simulink model "Trafo3"  (Simulink 6.5)
settings: Solver=ode23t  StartTime=0.0  StopTime=0.4  RelTol=1e-3
undefined symbols (not defined in the file): D1, Delta, powergui
libraries: powerlib_extras x12, powerlib x11
settings Model: Creator=RS  LastModifiedBy=RS

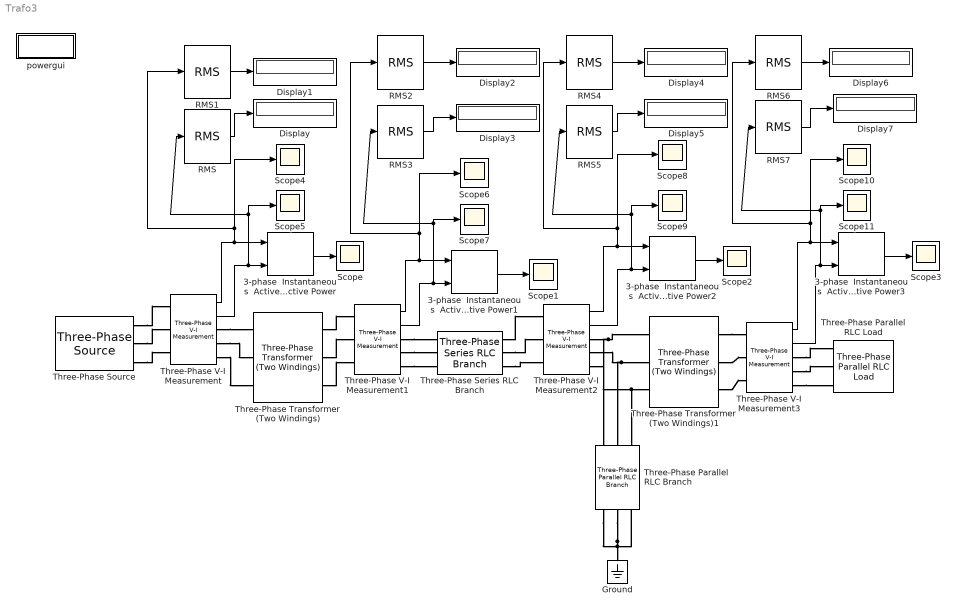
== system Trafo3 ==
  3-phase  Instantaneous  Active & Reactive Power{,1..3} (4 alike) : powerlib_extras/Measurements/3-phase  Instantaneous  Active & Reactive Power  DialogController=PMDialogs.PMDefaultMaskDlg  SystemSampleTime=-1
  Display{,1..7} (8 alike) : Display
  Ground : powerlib/Elements/Ground  Orientation=down  DialogController=PMDialogs.PMDefaultMaskDlg  PhysicalDomain=powersysdomain  SubClassName=unknown  LeftPortType=p1  RightPortType=p1  LConnTagsString=a
  RMS{,1..7} (8 alike) : powerlib_extras/Measurements/RMS  DialogController=PMDialogs.PMDefaultMaskDlg  SystemSampleTime=-1  f1=60
  Scope{,1..11} (12 alike) : Scope
      Scope settings: MaxDataPoints=10000000  SampleInput=on  SampleTime=10e-6
      Scope1 settings: MaxDataPoints=10000000  SampleInput=on  SampleTime=10e-6
      Scope10 settings: SaveName=ScopeData10  MaxDataPoints=10000000  SampleInput=on  SampleTime=10e-6
      Scope11 settings: SaveName=ScopeData11  MaxDataPoints=10000000  SampleInput=on  SampleTime=10e-6
      Scope2 settings: SaveName=ScopeData2  MaxDataPoints=10000000  SampleInput=on  SampleTime=10e-6
      Scope3 settings: YMin=-250000  YMax=3.25e+006  SaveName=ScopeData3  MaxDataPoints=10000000  SampleInput=on  SampleTime=10e-6
      Scope4 settings: SaveName=ScopeData4  MaxDataPoints=10000000  SampleInput=on  SampleTime=10e-6
      Scope5 settings: SaveName=ScopeData5  MaxDataPoints=10000000  SampleInput=on  SampleTime=10e-6
      Scope6 settings: SaveName=ScopeData6  MaxDataPoints=10000000  SampleInput=on  SampleTime=10e-6
      Scope7 settings: SaveName=ScopeData7  MaxDataPoints=10000000  SampleInput=on  SampleTime=10e-6
      Scope8 settings: SaveName=ScopeData8  MaxDataPoints=10000000  SampleInput=on  SampleTime=10e-6
      Scope9 settings: SaveName=ScopeData9  MaxDataPoints=10000000  SampleInput=on  SampleTime=10e-6
  Three-Phase Parallel RLC Branch : powerlib/Elements/Three-Phase Parallel RLC Branch  Orientation=down  DialogController=PMDialogs.PMDefaultMaskDlg  PhysicalDomain=powersysdomain  SubClassName=unknown  LeftPortType=p1  RightPortType=p1  LConnTagsString=A|B|C  RConnTagsString=A|B|C  BranchType=R  Resistance=10000000  Inductance=1e-3  Capacitance=1e-6  Measurements=None
  Three-Phase Parallel RLC Load : powerlib/Elements/Three-Phase Parallel RLC Load  DialogController=PMDialogs.PMDefaultMaskDlg  PhysicalDomain=powersysdomain  SubClassName=unknown  LeftPortType=p1  RightPortType=p1  LConnTagsString=A|B|C  Configuration=Y (grounded)  NominalVoltage=13200  NominalFrequency=60  ActivePower=3000000  InductivePower=0  CapacitivePower=0  Measurements=None
  Three-Phase Series RLC Branch : powerlib/Elements/Three-Phase Series RLC Branch  DialogController=PMDialogs.PMDefaultMaskDlg  PhysicalDomain=powersysdomain  SubClassName=unknown  LeftPortType=p1  RightPortType=p1  LConnTagsString=A|B|C  RConnTagsString=A|B|C  BranchType=RL  Resistance=7.3  Inductance=0.0483  Capacitance=1e-6  Measurements=None
  Three-Phase Transformer (Two Windings) : powerlib/Elements/Three-Phase Transformer (Two Windings)  DialogController=PMDialogs.PMDefaultMaskDlg  SystemSampleTime=-1  UNITS=SI  NominalPower="[ 3000000    60 ]"  Winding1Connection=Y  Winding1="[110000    20    0.42]"  Winding2Connection=Delta (D1)  Winding2="[33000  1.8     0.038]"  SetSaturation=off  Rm=99999999  Lm=99999999  Saturation=[0 0;0.66653 1910.3;277.72 2419.7]  Hysteresis=off  DataFile='hysteresis'  SetInitialFlux=off  InitialFluxes=[1273.5 -1273.5 1114.3]  Measurements=None  TransfoNumber=0  MoreParameters=off  BreakLoop=off  DataType=on
  Three-Phase Transformer (Two Windings)1 : powerlib/Elements/Three-Phase Transformer (Two Windings)  DialogController=PMDialogs.PMDefaultMaskDlg  SystemSampleTime=-1  UNITS=SI  NominalPower="[3000000    60 ]"  Winding1Connection=Delta (D1)  Winding1="[33000  1.8    0.026]"  Winding2Connection=Delta (D1)  Winding2="[13200    0.29    0.00416]"  SetSaturation=off  Rm=64821.4  Lm=18.9  Saturation=[0 0;8.571 148.55;3571.2 188.17]  Hysteresis=off  DataFile='hysteresis'  SetInitialFlux=off  InitialFluxes=[99.035 -99.035 86.655]  Measurements=None  TransfoNumber=0  MoreParameters=off  BreakLoop=off  DataType=on
  Three-Phase V-I Measurement{,1..3} (4 alike) : powerlib/Measurements/Three-Phase V-I Measurement  DialogController=PMDialogs.PMDefaultMaskDlg  SystemSampleTime=-1  VoltageMeasurement=phase-to-ground  SetLabelV=off  LabelV=Vabc  Vpu=off  CurrentMeasurement=yes  SetLabelI=off  LabelI=Iabc  Ipu=off  Pbase=100e6  Vbase=500e3  OutputType=Complex  PhasorSimulation=off  PSBequivalent=0
  Three-Phase Source : powerlib/Electrical Sources/Three-Phase Source  DialogController=PMDialogs.PMDefaultMaskDlg  SystemSampleTime=-1  Voltage=117000  PhaseAngle=0  Frequency=60  InternalConnection=Yg  SpecifyImpedance=off  Resistance=0.0001  Inductance=0.00001  ShortCircuitLevel=100e6  BaseVoltage=25e3  XRratio=7
  powergui : Subsystem  AncestorBlock=powerlib/powergui  InitFcn=powergui( 'InitFcn_Callback' , gcb , 0 , [ ] );  mask(PSB option menu block){SimulationMode=Continuous, SampleTime=50e-6, echomessages=off, RestoreLinks=warning, x0status=blocks, Frange=[0:2:500], Ylog=off, Xlog=on, ShowGrid=off, save=off, variable=ZData, structure=, ZoomFFT=on, StartTime=0.0, cycles=1, DisplayStyle=1, fundamental=60, FreqAxis=off, MaxFrequency=1000, frequencyindice=60, frequencyindicesteady=1, RmsSteady=1, display=off, Ts=0, frequency=60, methode=off, HookPort=off, Interpol=off}
      mask prompts: SimulationMode "Simulation mode"; SampleTime "Sample time Ts (when simulation mode is Discrete) (s)"; echomessages "Echo  Messages"; RestoreLinks "Restore disabled links"; x0status "Initial electrical states status"; Frange "Impedance tool: Frequency Range"; Ylog "Impedance tool: Log impedance"; Xlog "Impedance tool: log Frequency"; ShowGrid "Impedance tool: grid"; save "Impedance tool: Save Data To Workspace"; variable "Impedance tool: Variable Name"; structure "Structure Name (PSBFFTSCOPE)"; ZoomFFT "ZoomFFT (PSBFFTSCOPE)"; StartTime "Start Time (PSBFFTSCOPE)"; cycles "Cycles (PSBFFTSCOPE)"; DisplayStyle "Display style (PSBFFTSCOPE)"; fundamental "Fundamental (PSBFFTSCOPE)"; FreqAxis "Frequency Axis (PSBFFTSCOPE)"; MaxFrequency "Max Frequency (PSBFFTSCOPE)"; frequencyindice "Load flow frequency (Hz)"; frequencyindicesteady "Frequency indice (STEADYSTATE)"; RmsSteady "RMS display (STEADYSTATE)"; display "Display Results"; Ts "OBSOLETE 1"; frequency "Phasor frequency (Hz)"; methode "Phasor simulation"; HookPort "Hook port"; Interpol "Interpolate"
      mask init:
      | powerlibroot = which('powersysdomain');
      | PSBroot = powerlibroot(1:end-16);
      | %
      | switch SimulationMode
      | 	case 1
      | 		message=sprintf('Continuous');
      | 	case 2
      |         SampleTimeeval=evalin('base',SampleTime,'NaN');
      |         if isnan(SampleTimeeval)
      |             message=sprintf('Warning !!,\nUndefined sample time');
      |         else
      |             message=sprintf('Discrete,\nTs = %.4g s.',SampleTimeeval);
      |         end
      | 	case 3
      | 		message=sprintf('Phasors');
      | end
      | if strcmp(bdroot,'powerlib')
      |   message='powergui';
      | end
      | power_initmask();
      settings: CopyFcn=powergui( 'Copy_Callback' , gcb , 0 , [ ] );  ModelCloseFcn=powergui( 'CloseButton_Callback' , gcb , [ ] , [ ] );  PreSaveFcn=powergui( 'CloseButton_Callback' , gcb , [ ] , [ ] );  NameChangeFcn=powergui( 'NameChangeFcn_Callback' , gcb , 0 , [ ] );
      settings: DeleteFcn=|
      | powergui( 'Copy_Callback' , gcb , 1 , [ ] );
      | powergui( 'CloseButton_Callback' , gcb , [ ] , [ ] );
      settings: OpenFcn=|
      | if (power_openblockproxy ('secondary'))
      | powergui(gcb,'PM')
      | end;
      mask Help: web(psbhelp)
      mask StyleString: popup(Continuous|Discrete|Phasor),edit,checkbox,popup(yes|warning|no),popup(blocks|steady|zero),edit,checkbox,checkbox,checkbox,checkbox,edit,edit,checkbox,edit,edit,edit,edit,checkbox,edit,edit,edit,edit,checkbox,edit,edit,checkbox,checkbox,checkbox
      mask CallbackString: ||||||||||||||||||||||||||powergui('HookPort',[],[],gcb);|
      mask Display: disp(message)
  wires:
  Three-Phase V-I Measurement/1 -> 3-phase  Instantaneous  Active & Reactive Power/1, Scope4/1, RMS1/1
  Three-Phase V-I Measurement/2 -> 3-phase  Instantaneous  Active & Reactive Power/2, Scope5/1, RMS/1
  Three-Phase V-I Measurement1/1 -> 3-phase  Instantaneous  Active & Reactive Power1/1, Scope6/1, RMS2/1
  Three-Phase V-I Measurement1/2 -> 3-phase  Instantaneous  Active & Reactive Power1/2, Scope7/1, RMS3/1
  Three-Phase V-I Measurement2/1 -> 3-phase  Instantaneous  Active & Reactive Power2/1, Scope8/1, RMS4/1
  Three-Phase V-I Measurement2/2 -> 3-phase  Instantaneous  Active & Reactive Power2/2, Scope9/1, RMS5/1
  Three-Phase V-I Measurement3/1 -> 3-phase  Instantaneous  Active & Reactive Power3/1, Scope10/1, RMS6/1
  Three-Phase V-I Measurement3/2 -> 3-phase  Instantaneous  Active & Reactive Power3/2, Scope11/1, RMS7/1
  3-phase  Instantaneous  Active & Reactive Power3/1 -> Scope3/1
  3-phase  Instantaneous  Active & Reactive Power2/1 -> Scope2/1
  3-phase  Instantaneous  Active & Reactive Power1/1 -> Scope1/1
  3-phase  Instantaneous  Active & Reactive Power/1 -> Scope/1
  RMS/1 -> Display/1
  RMS1/1 -> Display1/1
  RMS2/1 -> Display2/1
  RMS3/1 -> Display3/1
  RMS4/1 -> Display4/1
  RMS5/1 -> Display5/1
  RMS6/1 -> Display6/1
  RMS7/1 -> Display7/1
  connections:
  Three-Phase Source/RConn1 -- Three-Phase V-I Measurement/LConn1
  Three-Phase Source/RConn2 -- Three-Phase V-I Measurement/LConn2
  Three-Phase Source/RConn3 -- Three-Phase V-I Measurement/LConn3
  Three-Phase V-I Measurement/RConn1 -- Three-Phase Transformer (Two Windings)/LConn1
  Three-Phase V-I Measurement/RConn2 -- Three-Phase Transformer (Two Windings)/LConn2
  Three-Phase V-I Measurement/RConn3 -- Three-Phase Transformer (Two Windings)/LConn3
  Three-Phase Transformer (Two Windings)/RConn1 -- Three-Phase V-I Measurement1/LConn1
  Three-Phase Transformer (Two Windings)/RConn2 -- Three-Phase V-I Measurement1/LConn2
  Three-Phase Transformer (Two Windings)/RConn3 -- Three-Phase V-I Measurement1/LConn3
  Three-Phase V-I Measurement1/RConn1 -- Three-Phase Series RLC Branch/LConn1
  Three-Phase V-I Measurement1/RConn2 -- Three-Phase Series RLC Branch/LConn2
  Three-Phase V-I Measurement1/RConn3 -- Three-Phase Series RLC Branch/LConn3
  Three-Phase Series RLC Branch/RConn1 -- Three-Phase V-I Measurement2/LConn1
  Three-Phase Series RLC Branch/RConn2 -- Three-Phase V-I Measurement2/LConn2
  Three-Phase Series RLC Branch/RConn3 -- Three-Phase V-I Measurement2/LConn3
  Three-Phase V-I Measurement2/RConn1 -- Three-Phase Transformer (Two Windings)1/LConn1 -- Three-Phase Parallel RLC Branch/LConn1
  Three-Phase V-I Measurement2/RConn2 -- Three-Phase Transformer (Two Windings)1/LConn2 -- Three-Phase Parallel RLC Branch/LConn2
  Three-Phase V-I Measurement2/RConn3 -- Three-Phase Transformer (Two Windings)1/LConn3 -- Three-Phase Parallel RLC Branch/LConn3
  Three-Phase Transformer (Two Windings)1/RConn1 -- Three-Phase V-I Measurement3/LConn1
  Three-Phase Transformer (Two Windings)1/RConn2 -- Three-Phase V-I Measurement3/LConn2
  Three-Phase Transformer (Two Windings)1/RConn3 -- Three-Phase V-I Measurement3/LConn3
  Three-Phase V-I Measurement3/RConn1 -- Three-Phase Parallel RLC Load/LConn1
  Three-Phase V-I Measurement3/RConn2 -- Three-Phase Parallel RLC Load/LConn2
  Three-Phase V-I Measurement3/RConn3 -- Three-Phase Parallel RLC Load/LConn3
  Three-Phase Parallel RLC Branch/RConn2 -- Three-Phase Parallel RLC Branch/RConn1 -- Three-Phase Parallel RLC Branch/RConn3 -- Ground/LConn1

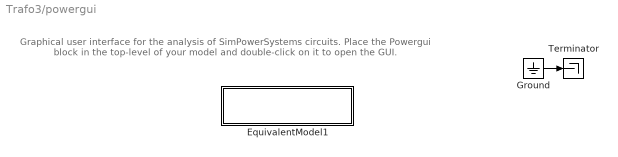
== system Trafo3/powergui ==
  note: Graphical user interface for the analysis of  SimPowerSystems circuits.
      | Place the Powergui block in the top-level of your model and double-click
      | on it to open the GUI.
  EquivalentModel1 : Subsystem
      mask init:
      | SPS = get_param(gcbh,'UserData');
      | if isempty(SPS)
      |     A=0;
      |     B=0;
      |     C=0;
      |     D=0;
      |     x0=0;
      | else
      | 	A=SPS.A;
      |     B=SPS.B;
      |     C=SPS.C;
      |     D=SPS.D;
      |     x0=SPS.x0;
      | end
      mask Display:
      | color('green')
      | disp('EQUIVALENT CIRCUIT')
  Ground : Ground
  Terminator : Terminator
  wires:
  Ground/1 -> Terminator/1

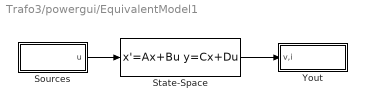
== system Trafo3/powergui/EquivalentModel1 ==
  Sources : Subsystem
  State-Space : StateSpace  A=A  B=B  C=C  D=D  X0=x0
  Yout : Subsystem
  wires:
  Sources/1(u) -> State-Space/1
  State-Space/1 -> Yout/1(v,i)

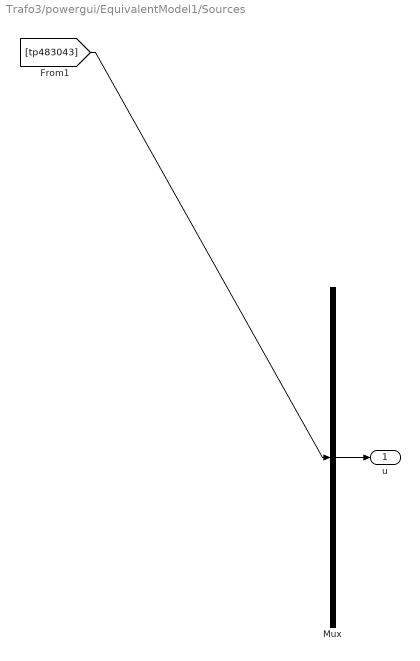
== system Trafo3/powergui/EquivalentModel1/Sources ==
  Mux : Mux  Inputs=1
  u : Outport
  wires:
  Mux/1 -> u/1
  [tp483043] -> Mux/1

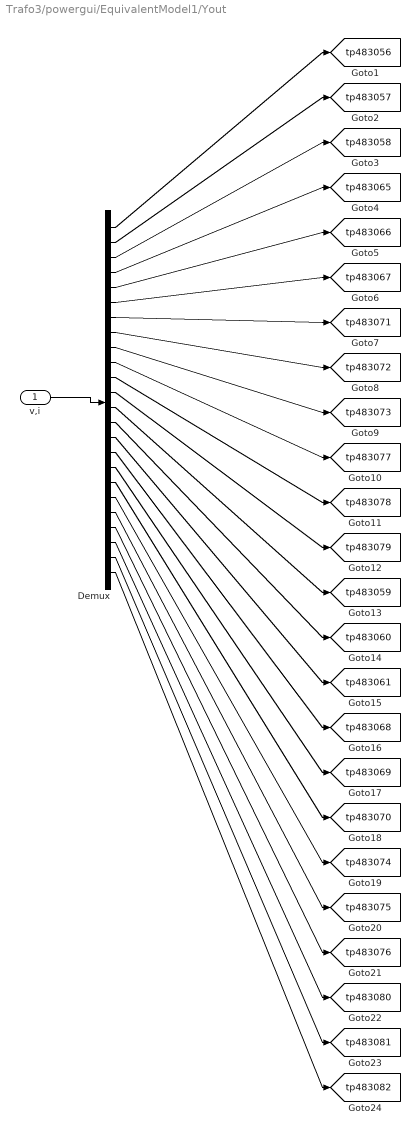
== system Trafo3/powergui/EquivalentModel1/Yout ==
  v,i : Inport
  Demux : Demux  Outputs=[1 1 1 1 1 1 1 1 1 1 1 1 1 1 1 1 1 1 1 1 1 1 1 1]
  tag scope: tp483056=global, tp483057=global, tp483058=global, tp483059=global, tp483060=global, tp483061=global, tp483065=global, tp483066=global, tp483067=global, tp483068=global, tp483069=global, tp483070=global, tp483071=global, tp483072=global, tp483073=global, tp483074=global, tp483075=global, tp483076=global, tp483077=global, tp483078=global, tp483079=global, tp483080=global, tp483081=global, tp483082=global
  wires:
  v,i/1 -> Demux/1
  Demux/1 -> [tp483056]
  Demux/2 -> [tp483057]
  Demux/3 -> [tp483058]
  Demux/4 -> [tp483065]
  Demux/5 -> [tp483066]
  Demux/6 -> [tp483067]
  Demux/7 -> [tp483071]
  Demux/8 -> [tp483072]
  Demux/9 -> [tp483073]
  Demux/10 -> [tp483077]
  Demux/11 -> [tp483078]
  Demux/12 -> [tp483079]
  Demux/13 -> [tp483059]
  Demux/14 -> [tp483060]
  Demux/15 -> [tp483061]
  Demux/16 -> [tp483068]
  Demux/17 -> [tp483069]
  Demux/18 -> [tp483070]
  Demux/19 -> [tp483074]
  Demux/20 -> [tp483075]
  Demux/21 -> [tp483076]
  Demux/22 -> [tp483080]
  Demux/23 -> [tp483081]
  Demux/24 -> [tp483082]
